simulink model "ADCS_onOrbit"  (R2024b)
settings: Solver=ode4  StartTime=0.0  StopTime=tspan  FixedStep=baseRate  RelTol=1e-3
values from neighbouring files (symbols this model uses):
  A_list = [10*30; 10*30; 10*10; 10*30; 10*30; 10*10] * 1e-04    [adcsInitializer.m]
  A_m = eye(3)    [adcsInitializer.m]
  A_w = eye(3)    [adcsInitializer.m]
  CD = 2.3    [adcsInitializer.m]
  COP = [xAxis/2   0          0 ... (first row only)    [adcsInitializer.m]
  dt = 1    [adcsInitializer.m]
  dYear = decyear(YYYY,MM,DD)    [adcsInitializer.m]
  eta = 0.3    [adcsInitializer.m]
  J_body = [ I_xx  I_xy  I_xz ... (first row only)    [adcsInitializer.m]
  JD0 = juliandate(YYYY,MM,DD,HH,MIN,SEC)    [adcsInitializer.m]
  m = 4    [adcsInitializer.m]
  mag_moment = [0.005; 0.005; 0.005]    [adcsInitializer.m]
  mode = mode(:)    [generateOutput.m]
  mu = 398600.4418    [adcsInitializer.m]    (also in montecarlo.m = mean(W,2))
  n_list = [1 0 0; 0 1 0; 0 0 1; -1 0 0; 0 -1 0; 0 0 -1]    [adcsInitializer.m]
  p = 0.00000451    (= 4.51e-06)    [adcsInitializer.m]
  R = blkdiag(sigma_S^2*eye(3), sigma_B^2*eye(3))    [adcsInitializer.m]
  rE = 6378.14    [adcsInitializer.m]
  sigma_b = deg2rad(0.04)/3600    [adcsInitializer.m]
  sigma_B = 0.001    [adcsInitializer.m]
  sigma_g = deg2rad(0.1)/sqrt(3600)    [adcsInitializer.m]
  sigma_S = deg2rad(0.01)    [adcsInitializer.m]
  T = 1    [adcsInitializer.m]
  wE = [0 0 15.04*(pi/180)*(1/3600)]    [adcsInitializer.m]
  wW_1 = 0    [adcsInitializer.m]
  wW_2 = 0    [adcsInitializer.m]
  wW_3 = 0    [adcsInitializer.m]
undefined symbols (not defined in the file or in its folder): DiscIntNeverNeededParam, J_wheels, K_d, K_p, K_w, n, period, q1_ini, q2_ini, q3_ini, q4_ini, r_I_ini, truevals, useFilter, v_I_ini, wB_1, wB_2, wB_3
libraries: simulink_extras x15, matrix_library x3
(part 2 of 2)

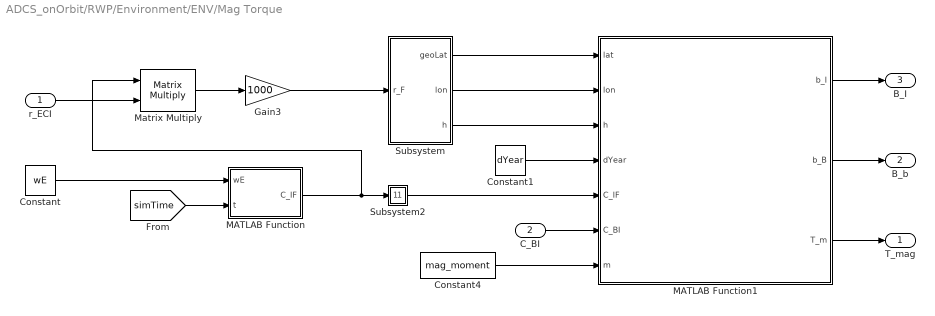
== system ADCS_onOrbit/RWP/Environment/ENV/Mag Torque ==
  r_ECI : Inport
  C_BI : Inport  Port=2
  Constant : Constant  Value=wE
  Constant1 : Constant  Value=dYear
  Constant4 : Constant  Value=mag_moment
  Gain3 : Gain  Gain=1000
  MATLAB Function : MATLAB Function  TreatAsAtomicUnit=on
  MATLAB Function1 : MATLAB Function  TreatAsAtomicUnit=on
  Matrix Multiply : Product  Multiplication=Matrix(*)
  Subsystem : Subsystem
  Subsystem2 : Subsystem
  T_mag : Outport
  B_b : Outport  Port=2
  B_I : Outport  Port=3
  wires:
  C_BI/1 -> MATLAB Function1/6(C_BI)
  Matrix Multiply/1 -> Gain3/1
  r_ECI/1 -> Matrix Multiply/2
  MATLAB Function/1(C_IF) -> Matrix Multiply/1, Subsystem2/1(In1)
  Constant/1 -> MATLAB Function/1(wE)
  [simTime] -> MATLAB Function/2(t)
  Subsystem/1(geoLat) -> MATLAB Function1/1(lat)
  Subsystem/2(lon) -> MATLAB Function1/2(lon)
  Constant1/1 -> MATLAB Function1/4(dYear)
  Constant4/1 -> MATLAB Function1/7(m)
  MATLAB Function1/1(b_I) -> B_I/1
  MATLAB Function1/2(b_B) -> B_b/1
  MATLAB Function1/3(T_m) -> T_mag/1
  Subsystem2/1(Out1) -> MATLAB Function1/5(C_IF)
  Gain3/1 -> Subsystem/1(r_F)
  Subsystem/3(h) -> MATLAB Function1/3(h)

== system ADCS_onOrbit/RWP/Environment/ENV/Solar Radiation Pressure ==
  C_BI : Inport
  s : Inport  Port=2
  MATLAB Function2 : MATLAB Function  TreatAsAtomicUnit=on
  T_SRP : Outport
  wires:
  MATLAB Function2/1(T_SRP) -> T_SRP/1
  C_BI/1 -> MATLAB Function2/2(C_BI)
  s/1 -> MATLAB Function2/1(r_sun)
  [inEclipse] -> MATLAB Function2/3(inEclipse)

== system ADCS_onOrbit/RWP/Environment/ENV/Mag Torque/Subsystem ==
  r_F : Inport
  Constant2 : Constant  Value=rE
  Gain : Gain  Gain=1000
  Geocentric to Geodetic Latitude : Geoc2Geod
  MATLAB Function2 : MATLAB Function  TreatAsAtomicUnit=on
  Scope : Scope
  geoLat : Outport
  lon : Outport  Port=2
  h : Outport  Port=3
  wires:
  MATLAB Function2/2(lon) -> lon/1
  Constant2/1 -> Gain/1, MATLAB Function2/2(rE)
  r_F/1 -> MATLAB Function2/1(r_F)
  MATLAB Function2/1(lat) -> Geocentric to Geodetic Latitude/1
  Geocentric to Geodetic Latitude/1 -> geoLat/1
  MATLAB Function2/3(h) -> Scope/1, h/1
  Gain/1 -> Geocentric to Geodetic Latitude/2

== system ADCS_onOrbit/RWP/Environment/ENV/Mag Torque/Subsystem2 ==
  In1 : Inport
  Out1 : Outport
  tag scope: C_IF=global
  wires:
  In1/1 -> [C_IF], Out1/1

== matlab function ADCS_onOrbit/GNC/Guidance/Error/MATLAB Function ==
  settings: updateMethod=DISCRETE  sampleTime=baseRate
  data: q_error input; theta_e output
function theta_e = pointing_error(q_error)

    q_error = q_error/norm(q_error);
    q4 = q_error(4);
    
    theta_e = rad2deg(2*acos(q4));

end

== matlab function ADCS_onOrbit/GNC/Guidance/Subsystem3/MATLAB Function1 ==
  data: q input; roll output; pitch output; yaw output
function [roll, pitch, yaw] = fcn(q)

    E = q(1:3);
    n = q(4);

    C_BI = (n^2 - E'*E) * eye(3) + 2*(E*E') - 2*n*skew(E);

    roll    = atan2(C_BI(2,3),C_BI(3,3));
    pitch   = -asin(C_BI(1,3));
    yaw     = atan2(C_BI(1,2),C_BI(1,1)); 


end

== matlab function ADCS_onOrbit/RWP/Orbit Propator/MATLAB Function2 ==
  settings: updateMethod=DISCRETE  sampleTime=baseRate
  data: r_S input; s output
function s = fcn(r_S)

s = r_S/norm(r_S);

== matlab function ADCS_onOrbit/RWP/Environment/ENV/Mag Torque/MATLAB Function1 ==
  settings: updateMethod=DISCRETE  sampleTime=1
  data: lat input; b_I output; lon input; h input; dYear input; C_IF input; C_BI input; m input; b_B output; T_m output
function [b_I, b_B, T_m] = fcn(lat, lon, h, dYear, C_IF, C_BI, m)

    coder.extrinsic('wrldmagm');
    
    % dYear = 2025.0;
    b = zeros(3,1);
    lat_geo = lat;

    m_skew = skew(m);
    
    % World Magnetic Model
    % [b, H, DEC, DIP, F] = wrldmagm(h, lat, lon, dYear,'Custom','WMM2025.COF');
    [b, H, DEC, DIP, F] = wrldmagm(h, lat, lon, dYear, 2020);

    % Conversion to go from NED to ECEF
    sLat = sind(lat_geo);
    cLat = cosd(lat_geo);

    sLon = sind(lon);
    cLon = cosd(lon);
 
    C_FN = [-sLat*cLon -sLat*sLon cLat; -sLon cLon 0; -cLat*cLon -cLat*sLon -sLat]';
    b_ECEF = C_FN * b;

    % Going from ECEF to ECI
    b_I = C_IF * b_ECEF;

    % Conversion to Body Frame
    b_B = C_BI * b_I;

    % Magnetic Torque
    T_m = m_skew * b_B * 1e-09;

end

== matlab function ADCS_onOrbit/SENS/Magnetometer/MATLAB Function ==
  settings: updateMethod=DISCRETE  sampleTime=baseRate
  data: meas input; y output; true input; set input
function y = fcn(meas, true, set)

y = (set ~= 0) * true + (set == 0) * meas;

== matlab function ADCS_onOrbit/SENS/Sun Sensor/MATLAB Function ==
  settings: updateMethod=DISCRETE  sampleTime=baseRate
  data: meas input; y output; true input; set input
function y = fcn(meas, true, set)

y = (set ~= 0) * true + (set == 0) * meas;

== matlab function ADCS_onOrbit/RWP/Nonlinear Spacecraft/Spacecraft Dynamics/MATLAB Function1 ==
  settings: updateMethod=DISCRETE  sampleTime=baseRate
  data: h_tot input; T_b input; h_tot_dot output; h_w input; w_b output; J_body parameter; A_w parameter
function [h_tot_dot, w_b] = dynamics(h_tot, T_b, h_w, J_body, A_w)

% Nimish Dhawan 2025

% T_b : net body torque (ext + MTQ - wheel torque on body)      [3x1]
% J     : body inertia                                          [3x3]
% A_w   : wheel axis matrix (columns = wheel axes, body frame)  [3x3]
% h_w   : wheel angular momentum                                [3x1]
% h_tot : current total angular momentum of SC (state)          [3x1]

% ---- omega from momentum ----
w_b = J_body \ (h_tot - A_w * h_w);       

% ---- h_tot dynamics ----
h_tot_dot = T_b - skew(w_b) * h_tot;

end

== matlab function ADCS_onOrbit/RWP/Nonlinear Spacecraft/Spacecraft Kinematics/MATLAB Function1 ==
  settings: updateMethod=DISCRETE  sampleTime=baseRate
  data: q input; q_dot output; w input
function q_dot = kinematics(q, w)

% Nimish Dhawan 2025
% Input: 
% q = quaternion (4x1) [scalar last]
% w = angular velocity of s/c (3x1) [SBF]

E   = q(1:3);
Eta = q(4);

E_dot   = 0.5 * (Eta*eye(3) + skew(E)) * w;
Eta_dot = -0.5 * (E' * w); 

q_dot = [E_dot; Eta_dot];

end

== matlab function ADCS_onOrbit/RWP/Nonlinear Spacecraft/Spacecraft Kinematics/Quaternion Normalize1 ==
  settings: updateMethod=DISCRETE  sampleTime=baseRate
  data: q input; q_norm output
function q_norm = q_normalize(q)

q_norm = q/norm(q);

== matlab function ADCS_onOrbit/RWP/Orbit Propator/Two Body/MATLAB Function1 ==
  settings: updateMethod=DISCRETE  sampleTime=baseRate
  data: r_I input; a_I output; mu input
function a_I = fcn(r_I, mu)

a_I = r_I .* (-mu / (norm(r_I)^3));

end

== matlab function ADCS_onOrbit/RWP/Orbit Propator/Two Body/MATLAB Function3 ==
  settings: updateMethod=DISCRETE  sampleTime=baseRate
  data: r input; a_j2 output; mu input; rE input
function a_j2 = J2_perturbation(r, mu, rE)

    J2 = 1.08263e-3;

    x = r(1); y = r(2); z = r(3);
    r_norm = norm(r);

    factor = -(3/2) * J2 * mu * rE^2 / r_norm^5;
    zx2_r2 = 5*z^2 / r_norm^2;

    a_j2 = factor * [
        x * (1 - zx2_r2);
        y * (1 - zx2_r2);
        z * (3 - zx2_r2)
    ];
    
end

== matlab function ADCS_onOrbit/RWP/Orbit Propator/MATLAB Function ==
  settings: updateMethod=DISCRETE  sampleTime=baseRate
  data: q input; C_BI output
function C_BI = QUAT2DCM(q)

% Nimish Dhawan
% 2025

%%%%%%%%%%%%%%%%%%%%%%%%%%%%%%%%%%%%%%%%%%%%%%%%%%%%%%%%%%%%%%%%%%%%%%%%%
% Input(s)
%%%%%%%%%%%%%%%%%%%%%%%%%%%%%%%%%%%%%%%%%%%%%%%%%%%%%%%%%%%%%%%%%%%%%%%%%
% q (4x1): Quaternion

%%%%%%%%%%%%%%%%%%%%%%%%%%%%%%%%%%%%%%%%%%%%%%%%%%%%%%%%%%%%%%%%%%%%%%%%%
% Output(s)
%%%%%%%%%%%%%%%%%%%%%%%%%%%%%%%%%%%%%%%%%%%%%%%%%%%%%%%%%%%%%%%%%%%%%%%%%
% C_BI (3x3): Rotation matrix to go from ECI to Body Fixed Frame

E = q(1:3);
Eta = q(4);

C_BI = (Eta^2-E'*E)*eye(3) + 2*(E*E') - 2*Eta*skew(E);

== matlab function ADCS_onOrbit/ACT/Wheels + Magnetorquers/Wheel 1/MATLAB Function1 ==
  settings: updateMethod=DISCRETE  sampleTime=baseRate
  data: h_wi output; w_wi output; J_w input; h_w input; wB input; A_w input
function [h_wi, w_wi] = fcn(J_w, h_w, wB, A_w)

% Nimish Dhawan 2025

i       = 1;      % Wheel No.


J_inv   = 1 / J_w;
Aw_i    = A_w(:,i);
h_wi    = h_w ;

w_wi = (J_inv*h_wi) * Aw_i;

end

== matlab function ADCS_onOrbit/ACT/Wheels + Magnetorquers/Wheel 2/MATLAB Function1 ==
  settings: updateMethod=DISCRETE  sampleTime=baseRate
  data: h_wi output; w_wi output; J_w input; h_w input; wB input; A_w input
function [h_wi, w_wi] = fcn(J_w, h_w, wB, A_w)

% Nimish Dhawan 2025

i       = 2;      % Wheel No.

J_inv   = 1 / J_w;
Aw_i    = [A_w(:,i)];
h_wi    = h_w ;

w_wi = (J_inv*h_wi) * Aw_i;

end

== matlab function ADCS_onOrbit/RWP/Environment/MATLAB Function ==
  settings: updateMethod=DISCRETE  sampleTime=baseRate
  data: u input; y output
function y = magnitude(u)

y = norm(u);

== matlab function ADCS_onOrbit/ACT/Wheels + Magnetorquers/Wheel 3/MATLAB Function1 ==
  settings: updateMethod=DISCRETE  sampleTime=baseRate
  data: h_wi output; w_wi output; J_w input; h_w input; wB input; A_w input
function [h_wi, w_wi] = fcn(J_w, h_w, wB, A_w)

% Nimish Dhawan 2025

i       = 3;      % Wheel No.

J_inv   = 1 / J_w;
Aw_i    = [A_w(:,i)];
h_wi    = h_w ;

w_wi = (J_inv*h_wi) * Aw_i;

end

== matlab function ADCS_onOrbit/RWP/Environment/ENV/Gravity Gradient/MATLAB Function3 ==
  settings: updateMethod=DISCRETE  sampleTime=1
  data: r_I input; J input; mu input; C_BI input; T_g output
function T_g = fcn(r_I, J, mu, C_BI)

r_B = C_BI * r_I;
r = norm(r_I);

T_g = (3*mu/r^5) * skew(r_B) * J * r_B;

== matlab function ADCS_onOrbit/ACT/Wheels + Magnetorquers/Reaction Wheel Power/MATLAB Function3 ==
  data: Tc input; Prw output; h_W input; Ptotal output; P_pre input
function [Prw, Ptotal]= fcn(Tc, h_W, P_pre)

% Nimish Dhawan
% Reaction wheel power consumption as given in "Comarison of Control Moment
% Gyros and Reaction Wheels for Small Earth-Observing Satellites


% Eq. 3
alpha = 0.47;     % empirical exponent
k2    = 4.51;     % empirical coeff

Prw = 1000.*abs(Tc) + k2.*(abs(h_W).^(alpha));   % per-wheel power [W]
Ptotal = (P_pre + Prw); 

end

== matlab function ADCS_onOrbit/GNC/Guidance/Attitude Guidance ==
  settings: updateMethod=DISCRETE  sampleTime=baseRate
  data: q_prev input; opMode input; s_i input; r input; v input; C_IF input; q output; w output; mode output; n parameter; rE parameter; CQI output
function [q, w, mode, CQI] = fcn(q_prev, opMode, s_i, r, v, C_IF, n, rE)


    option = opMode;
    q = zeros(4,1);
    w = zeros(3,1);
    CQI = zeros(3,3);
    mode = 0;

    % Manual override modes
    % For mission mode, detumble mode, desaturation mode and safemode
    if option ~= 1 && option ~= 2 && option ~= 3
        [q, w] = nadir(r, v, n, q_prev);
        mode = 0;

    % For comms mode
    elseif option == 3
        [q, w] = gnd(C_IF, rE, r, v, q_prev);
       
    % Idle mode
    elseif option == 1
        [q, w] = sun(s_i);
        mode = 1;
    end

    CQI = rpy(r, v);
end

%%
function [q_nadir, w_nadir] = nadir(r, v, n, q_prev)

    C_BI = rpy(r, v);

    q = CBI2quat(C_BI');
    q_nadir = continuity(q, q_prev);
    w_nadir = [0; -n; 0];
end

%%
function [q_sun, w_sun] = sun(s_i)
    % coder.extrinsic('dcm2quat');
    % Ecliptic north pole
    epsilon = deg2rad(23.44);  % Obliquity of the ecliptic
    n_ecl = [0; -sin(epsilon); cos(epsilon)];

    x_b = s_i / norm(s_i);
    z_b = n_ecl - dot(n_ecl, x_b) * x_b; % Gram-Schmidt orthogonalization
    z_b = z_b / norm(z_b); 
    if dot(z_b, n_ecl) < 0
        z_b = -z_b; 
    end
    y_b = cross(z_b, x_b);
    
    C1 = [x_b y_b z_b];   

    theta = deg2rad(45);

    Rz = [cos(theta), sin(theta), 0;
          -sin(theta), cos(theta), 0;
          0,           0,          1];
    
    C_BI = C1 * Rz;
    q = r2quat(C_BI);
    % q_sun = continuity(q, q_prev);
    % q_sun = [q(2:4);q(1)];
    q_sun = q;
    w_sun = [0;0;0];

end

%%
function [q_gnd, w_gnd] = gnd(C_IF, rE, r, v, q_prev)
    dt = 1;

    target_lat = 45.3848;
    target_lon = - 75.6974;

    lat = deg2rad(target_lat);
    lon = deg2rad(target_lon);
    
    x_F= rE * cos(lat) * cos(lon);
    y_F= rE * cos(lat) * sin(lon);
    z_F= rE * sin(lat);
    
    r_target_I = C_IF * [x_F; y_F; z_F];
    los = r - r_target_I;
    los = los / norm(los);
    
    z_orb = los;

    y_orb = cross(v, r) / norm(cross(v,r)); % orbit normal
    y_orb = y_orb / norm(y_orb);

    x_orb = cross(y_orb, z_orb); 
    x_orb = x_orb / norm(x_orb);
    
    C_BI = [x_orb, y_orb, z_orb];

    q = CBI2quat(C_BI);
    q_gnd = continuity(q, q_prev);
    q_dot = (q_gnd - q_prev)/dt;
    E = q_gnd(1:3);
    n = q_gnd(4);
    Edot = q_dot(1:3);
    w_gnd = (2/n) * (n^2*eye(3) - n*skew(E) + (E*E'))*Edot; 
end

%%
function CQI = rpy(r, v)
    z_orb = - r / norm(r);                  % nadir
    y_orb = cross(v, r) / norm(cross(v,r)); % orbit normal
    y_orb = y_orb / norm(y_orb);

    x_orb = cross(y_orb, z_orb); 
    x_orb = x_orb / norm(x_orb);

    CQI = [x_orb, y_orb, z_orb]';
end

%%
function q = r2quat(DCM)
    A = DCM;
    q = zeros(4,1); % [q1; q2; q3; q4] — vector-first

    tr = trace(A);

    if tr > 0
        S = sqrt(tr + 1.0) * 2; % S = 4*q4
        q(4) = 0.25 * S;
        q(1) = (A(3,2) - A(2,3)) / S;
        q(2) = (A(1,3) - A(3,1)) / S;
        q(3) = (A(2,1) - A(1,2)) / S;
    elseif (A(1,1) > A(2,2)) && (A(1,1) > A(3,3))
        S = sqrt(1.0 + A(1,1) - A(2,2) - A(3,3)) * 2; % S = 4*q1
        q(1) = 0.25 * S;
        q(2) = (A(1,2) + A(2,1)) / S;
        q(3) = (A(1,3) + A(3,1)) / S;
        q(4) = (A(3,2) - A(2,3)) / S;
    elseif (A(2,2) > A(3,3))
        S = sqrt(1.0 + A(2,2) - A(1,1) - A(3,3)) * 2; % S = 4*q2
        q(1) = (A(1,2) + A(2,1)) / S;
        q(2) = 0.25 * S;
        q(3) = (A(2,3) + A(3,2)) / S;
        q(4) = (A(1,3) - A(3,1)) / S;
    else
        S = sqrt(1.0 + A(3,3) - A(1,1) - A(2,2)) * 2; % S = 4*q3
        q(1) = (A(1,3) + A(3,1)) / S;
        q(2) = (A(2,3) + A(3,2)) / S;
        q(3) = 0.25 * S;
        q(4) = (A(2,1) - A(1,2)) / S;
    end

    q = q / norm(q); % normalize
end

== matlab function ADCS_onOrbit/RWP/Environment/ENV/Drag/Atmosphere Model ==
  settings: updateMethod=DISCRETE  sampleTime=baseRate
  data: rho output; r input; rE input
function rho = atmosphere(r, rE)

    z = norm(r)-rE;        % Altitude (km) 
    
    if 400 <= z && z < 450
        rho0 = 3.275e-12;
        h0   = 400;
        H    = 58.515;
    elseif 450 <= z && z < 500
        rho0 = 1.585e-12;   % kg/m³
        h0   = 450;   % km
        H    = 60.828;  % km
    elseif 500 <= z && z < 600
        rho0 = 6.967e-13;   % kg/m³
        h0   = 500;   % km
        H    = 63.822;  % km
    elseif 600 <= z && z < 700
        rho0 = 1.454e-13;
        h0   = 600;
        H    = 71.835;
    elseif 700 <= z && z < 800
        rho0 = 3.614e-14;
        h0   = 700;
        H    = 88.667;
    else
        rho0 = 1.170e-14;
        h0   = 800;
        H    = 124.64;
    end

    rho = rho0 * exp(-(z-h0)/H);    % in kg/m³

end

== matlab function ADCS_onOrbit/RWP/Environment/ENV/Drag/Drag Torque ==
  settings: updateMethod=DISCRETE  sampleTime=baseRate
  data: v_RI input; C_BI input; A_list input; n_list input; COP_B input; CD input; T_atm output; rho input; a_drag output; m input
function [T_atm, a_drag] = drag_torque(v_RI, C_BI, A_list, n_list, COP_B, CD, rho, m)

    v_RI_hat = v_RI / norm(v_RI);     
    v_RI_mag = norm(v_RI);            
    T_atm = [0; 0; 0];
    F_drag = [0; 0; 0];
    a_drag = [0; 0; 0];

    for k = 1:length(A_list)
        n_k = n_list(k, :).';         
        A_k = A_list(k);              

        cos_alpha_k = dot(n_k, C_BI * v_RI_hat);

        if cos_alpha_k > 0
            F_k = - 0.5 * rho * CD * A_k * v_RI_mag^2 * cos_alpha_k * v_RI_hat;
        else 
            F_k = [0; 0; 0];
        end
        F_drag = F_drag + F_k;
        a_drag = F_drag/m;

        F_k_B = C_BI * F_k;
        COP_B_k = COP_B(k, :).';
        T_k = cross(COP_B_k, F_k_B);
        T_atm = T_atm + T_k;
    end

end

== matlab function ADCS_onOrbit/TTC/RES/MATLAB Function ==
  data: u input; y output
function y = magnitude(u)

y = norm(u);

== matlab function ADCS_onOrbit/RWP/Environment/ENV/Drag/skew symmetric ==
  settings: updateMethod=DISCRETE  sampleTime=baseRate
  data: M input; skew output
function skew = skew_matrix(M)

    skew = [0 M(3) -M(2)
            -M(3) 0 M(1)
            M(2) -M(1) 0];

end

== matlab function ADCS_onOrbit/GNC/Navigation/MEKF/MEKF ==
  settings: updateMethod=DISCRETE  sampleTime=baseRate
  data: x_pre input; w_meas input; q_triad input; y input; useFilter input; q_est output; b_est output; P_pre input; P_est output; sigma_g parameter; sigma_b parameter; dt parameter; R parameter
function [q_est, b_est, P_est] = est(x_pre, w_meas, q_triad, y, useFilter , P_pre, sigma_g, sigma_b, ...
dt, R)

q_pre = x_pre(1:4);
b_pre = x_pre(5:7);

% Simulink acting out badly and thinking w_meas is 9x1
b_pre = reshape(b_pre, [3,1]);
w_meas = w_meas(1:3);   

s_I = y(1:3);
s_B = y(7:9);
b_I = y(4:6);
b_B = y(10:12);

if useFilter ~= 0
    [q_est, b_est, P_est] = mekf(q_pre, w_meas, b_pre, dt, s_I, ...
                                b_I, s_B, b_B, R, sigma_g, sigma_b, P_pre);
else
    q_est = q_triad;
    b_est = zeros(3,1);
    P_est = zeros(6,6);
end

end

== matlab function ADCS_onOrbit/RWP/Orbit Propator/Eclipse Detection/MATLAB Function3 ==
  settings: updateMethod=DISCRETE  sampleTime=baseRate
  data: R_s input; eclipse_entry output; r_sat input; r_E input; was_in_eclipse input; eclipse_exit output; is_in_eclipse output
function [eclipse_entry, eclipse_exit, is_in_eclipse] = fcn(R_s, r_sat, r_E, was_in_eclipse)

    % Convert input to numeric (if it came in as logical)
    if was_in_eclipse
        was = 1;
    else
        was = 0;
    end

    % Normalize sun vector
    s_hat = R_s / norm(R_s);

    % Projection of satellite position onto sun vector
    proj = dot(r_sat, s_hat);
    closest_point = proj * s_hat;

    % Perpendicular distance from Earth center to Sun-sat line
    d = norm(r_sat - closest_point);

    % Check if satellite is in eclipse
    if (d < r_E) && (proj < 0)
        is_in_eclipse = 1;
    else
        is_in_eclipse = 0;
    end

    % Detect eclipse entry
    if (was == 0) && (is_in_eclipse == 1)
        eclipse_entry = 1;
    else
        eclipse_entry = 0;
    end

    % Detect eclipse exit
    if (was == 1) && (is_in_eclipse == 0)
        eclipse_exit = 1;
    else
        eclipse_exit = 0;
    end

end

== matlab function ADCS_onOrbit/SENS/Gyroscope/MATLAB Function1 ==
  settings: updateMethod=DISCRETE  sampleTime=baseRate
  data: w_sc input; w_meas output; bias input; noise input
function w_meas = fcn(w_sc, bias, noise)

rand_w = noise .* ones(3,1);
bias   = bias .* ones(3,1);

w_meas = w_sc + bias + rand_w;

== matlab function ADCS_onOrbit/GNC/Navigation/Subsystem1/MATLAB Function2 ==
  data: q input; roll output; pitch output; yaw output; C_QI input
function [roll, pitch, yaw] = fcn(q, C_QI)

    E = q(1:3);
    n = q(4);

    C_BI = (n^2 - E'*E) * eye(3) + 2*(E*E') - 2*n*skew(E);
    C_BQ = C_BI * C_QI';
    
    roll    = atan2(C_BQ(2,3),C_BQ(3,3));
    pitch   = -asin(C_BQ(1,3));
    yaw     = atan2(C_BQ(1,2),C_BQ(1,1));

end

== matlab function ADCS_onOrbit/SENS/Gyroscope/MATLAB Function2 ==
  data: true input; meas input; y output; set input
function y = fcn(true, meas, set)

y = (set ~= 0) * true + (set == 0) * meas;

== matlab function ADCS_onOrbit/RWP/Environment/ENV/Mag Torque/Subsystem/MATLAB Function2 ==
  data: r_F input; lat output; lon output; rE input; h output
function [lat, lon, h] = fcn(r_F, rE)

r = norm(r_F);

lat = asind(r_F(3)/r);

if r_F(2)/r > 0
    lon = acosd(r_F(1)/(r*cosd(lat)));
else
    lon = 360 - acosd(r_F(1)/(r*cosd(lat)));
end

h = r - rE*1000;

end

== matlab function ADCS_onOrbit/ACT/Wheels + Magnetorquers/MATLAB Function ==
  settings: updateMethod=DISCRETE  sampleTime=baseRate
  data: T_c input; T_cmd output; wheelsEnabled input
function T_cmd = fcn(T_c, wheelsEnabled)

if wheelsEnabled == 1
    T_cmd = T_c;
else
    T_cmd = [0; 0; 0];
end

end

== matlab function ADCS_onOrbit/RWP/Environment/ENV/Mag Torque/MATLAB Function ==
  data: wE input; C_IF output; t input
function C_IF = fcn(wE, t)

    theta = wE(3) * t;

    C_IF = [cos(theta) sin(theta) 0; -sin(theta) cos(theta) 0; 0 0 1]';

end

== matlab function ADCS_onOrbit/RWP/Environment/ENV/Solar Radiation Pressure/MATLAB Function2 ==
  settings: updateMethod=DISCRETE  sampleTime=baseRate
  data: r_sun input; T_SRP output; C_BI input; inEclipse input; p parameter; eta parameter; A_list parameter; n_list parameter; COP parameter
function T_SRP = srpT(r_sun, C_BI, inEclipse, p, eta, A_list, n_list, COP)

    T_SRP = [0; 0; 0];
    r_sun = r_sun(:);  

    for k = 1:length(A_list)
        n_k = n_list(k, :)';          % column vector (3x1)
        A_k = A_list(k);              % scalar area

        cos_alpha_k = dot(n_k, C_BI * r_sun);  

        if cos_alpha_k > 0 && inEclipse == 0
            F_srp_k = -p * A_k * eta * cos_alpha_k * r_sun;  
        else
            F_srp_k = [0; 0; 0];
        end

        F_srp_k_B = C_BI * F_srp_k;
        COP_k = COP(k, :)';
        T_SRP_k = cross(COP_k, F_srp_k_B);

        T_SRP = T_SRP + T_SRP_k;
    end

end

== matlab function ADCS_onOrbit/GNC/Navigation/TRIAD Determination/MATLAB Function1 ==
  settings: updateMethod=DISCRETE  sampleTime=baseRate
  data: s_I input; q_triad output; m_I input; s_b input; m_b input; q_prev input
function q_triad = fcn(s_I, m_I, s_b, m_b, q_prev)

% Normalizing vectors
sI = s_I/norm(s_I);
sB = s_b/norm(s_b);
mI = m_I/norm(m_I);
mB = m_b/norm(m_b);

% Determining M_I 
r1 = sI;
r2 = skew(sI)*mI/norm(skew(sI)*mI);
r3 = skew(r1) * r2;
MI = [r1, r2, r3];

% Determining M_B
s1 = sB;
s2 = skew(sB)*mB/norm(skew(sB)*mB);
s3 = skew(s1) * s2;

MB = [s1, s2, s3]; 

C_BI = MB * MI';

q = CBI2quat(C_BI);
q_triad = continuity(q, q_prev);

end

%%

== matlab function ADCS_onOrbit/SENS/Gyroscope/MATLAB Function ==
  settings: updateMethod=DISCRETE  sampleTime=baseRate
  data: biasDot output; noise input
function biasDot = fcn(noise)

bias_noise = noise.*[1;1;1];

biasDot = bias_noise;

== matlab function ADCS_onOrbit/GNC/Control/Controller ==
  settings: updateMethod=DISCRETE  sampleTime=baseRate
  data: opMode input; t input; T_w output; B_meas input; w input; q_error input; w_error input; h_w input; M output; period parameter; J_body parameter; K_p parameter; K_d parameter; K_w parameter; m_pre input; m output
function [T_w, M, m] = fcn(opMode ,t, B_meas, w, q_error, w_error, h_w, period, J_body, K_p, K_d, K_w, m_pre)

T_w = [0; 0; 0];
M = [0; 0; 0];
w_skew = skew(w);

% Modified PD control
if opMode ~= 4 && opMode ~= 5 && opMode ~= 6 && opMode ~= 7 && opMode ~= 8

    % Gain Scheduling
    theta_e = 2*atan2(norm(q_error(1:3)), q_error(4));
    wr = norm(w_error);

    Kd0 = diag(K_d*ones(3,1));
    Kp0 = diag(K_p*ones(3,1));

    % Kd0 = diag([0.01, 0.025, 0.01]);
    % Kp0 = diag([0.000125/2, 0.000125, 0.000125/2])./2;

    e1 = deg2rad(1.0);
    e2 = deg2rad(3.0);
    w1 = deg2rad(0.05);
    w2 = deg2rad(0.1);

    % alpha_p = (theta_e < e1)*0.6 + (theta_e >= e1 && theta_e < e2)*5.0 + (theta_e >= e2)*1.6;
    % alpha_d = (wr < w1)*0.9 + (wr >= w1 && wr < w2)*1.2 + (wr >= w2)*1.6;

    alpha_p = (theta_e < e1)*0.6 + (theta_e >= e1 && theta_e < e2 && opMode == 0)*5.0 + ...
                (theta_e >= e1 && theta_e < e2 && opMode == 1)*0.2 + (theta_e >= e2)*1;
    alpha_d = (wr < w1)*0.9 + (wr >= w1 && wr < w2)*1.2 + (wr >= w2)*2;

    if wr >= w2
        alpha_p = 0.7*alpha_p;
        alpha_d = 1.3*alpha_d;
    end

    alpha_p = min(max(alpha_p,0.0),2.5);
    alpha_d = min(max(alpha_d,0.5),3.0);

    K_p = alpha_p*Kp0;
    K_d = alpha_d*Kd0;
        
    % K_d = diag([0.01, 0.025, 0.01]);
    % K_p = diag([0.000125/2, 0.000125, 0.000125/2])./2;

    % Control algorithm
    T_w = w_skew * J_body * w + K_p * eye(3) * q_error(1:3) + K_d * eye(3) * w_error;
    m = m_pre;

% B-dot 
elseif opMode == 8
    M = -K_w * skew(B_meas) * w;
    m = m_pre;

% No control - Safe mode and LEOP
elseif opMode == 6 || opMode == 7
    T_w = [0; 0; 0];
    M = [0; 0; 0];
    m = m_pre;

% Desaturation (incomplete)
elseif opMode == 5
    % Trigger for dumping
    if t < (12*period) && t > (10*period) % Create a proper autonomous trigger for dumping
        k_desat = -0.0005;
    else
        k_desat = 0;
    end

    % Controller gains
    K_p = 5e-4;
    K_d = 5e-05;
    
    % Desired wheel momentum [h_w1; h_w2; h_w3]
    h_wn = [0; 0; 0];
    B2 = norm(B_meas)^2;

    % Control algorithm
    T_ctrl = w_skew * J_body * w + K_p * eye(3) * q_error(1:3) + K_d * eye(3) * w_error;
    M_dump = (k_desat/B2) * (cross(B_meas, (h_w - h_wn))); 
    % T_dump = cross(M_dump, B_meas);

    T_w = T_ctrl;
    M = M_dump;
    % T_mag = T_dump;
    % 
    % M = (1/B2) * cross(B_meas, T_mag);
    m = m_pre;

% Simple Bdot Detumble (works)
elseif opMode == 4
    [T_w, M, m] = detumble(w, J_body, w_skew, q_error, K_p, K_d, K_w, w_error, B_meas, m_pre);

else
    % unknown opMode (or NaN) -> safe outputs
    T_w = [0;0;0];
    M   = [0;0;0];
    m   = 0;

end

end

%%
function [T_w, M, m] = detumble(w, J_body, w_skew, q_error, K_p, K_d, K_w, w_error, B_meas, m_pre)
% Latch doesnt work :(
    wr = norm(w);
    if m_pre ~= 1
        Kw0 = K_w;
        alpha = (wr > deg2rad(1)) * 5 + (wr <= deg2rad(1)) * 10;
        Kw = alpha*Kw0;
        M = - Kw * skew(B_meas) * w;
        T_w = [0; 0; 0];
        if wr < 0.01
            m = 1;
        else
            m = 0; 
        end
    elseif m_pre == 1  %wr < deg2rad(0.5) &&
        T_w = w_skew * J_body * w + K_p * eye(3) * q_error(1:3) + K_d * eye(3) * w_error;
        M = [0; 0; 0]; 
        m = 1;
    else
        T_w = [0; 0; 0];
        M = [0; 0; 0]; 
        m = 0;
    end

end

== matlab function ADCS_onOrbit/ACT/Wheels + Magnetorquers/Magnetorquer 1/skew symmetric ==
  data: M input; skew output
function skew = skew_matrix(M)

    skew = [0 M(3) -M(2)
            -M(3) 0 M(1)
            M(2) -M(1) 0];

end

== matlab function ADCS_onOrbit/ACT/Wheels + Magnetorquers/Magnetorquer 2/skew symmetric ==
  data: M input; skew output
function skew = skew_matrix(M)

    skew = [0 M(3) -M(2)
            -M(3) 0 M(1)
            M(2) -M(1) 0];

end

== matlab function ADCS_onOrbit/RWP/Nonlinear Spacecraft/Subsystem/MATLAB Function2 ==
  data: q input; roll output; pitch output; yaw output; C_QI input
function [roll, pitch, yaw] = fcn(q, C_QI)

    E = q(1:3);
    n = q(4);

    C_BI = (n^2 - E'*E) * eye(3) + 2*(E*E') - 2*n*skew(E);
    C_BQ = C_BI * C_QI';
    
    roll    = atan2(C_BQ(2,3),C_BQ(3,3));
    pitch   = -asin(C_BQ(1,3));
    yaw     = atan2(C_BQ(1,2),C_BQ(1,1));

end

== matlab function ADCS_onOrbit/ACT/Wheels + Magnetorquers/Magnetorquer 3/skew symmetric ==
  data: M input; skew output
function skew = skew_matrix(M)

    skew = [0 M(3) -M(2)
            -M(3) 0 M(1)
            M(2) -M(1) 0];

end

== matlab function ADCS_onOrbit/ACT/Wheels + Magnetorquers/MATLAB Function1 ==
  settings: updateMethod=DISCRETE  sampleTime=baseRate
  data: M_c input; M_cmd output; rodsEnable input
function M_cmd = fcn(M_c, rodsEnable)

if rodsEnable == 1
    M_cmd = M_c;
else
    M_cmd = [0; 0; 0];
end

end

== matlab function ADCS_onOrbit/GNC/Navigation/MATLAB Function ==
  settings: updateMethod=DISCRETE  sampleTime=baseRate
  data: u input; y output
function y = fcn(u)

y = norm(u);

== matlab function ADCS_onOrbit/TTC/MATLAB Function ==
  settings: updateMethod=DISCRETE  sampleTime=baseRate
  data: internal input; mode output; fromTable input; wheelsEnable output; rodsEnable output
function [mode, wheelsEnable, rodsEnable] = fcn(internal, fromTable)

if internal ~= 2
    mode = internal;
    wheelsEnable    = 1;
    rodsEnable      = 1;
else
    mode            = fromTable(1);
    wheelsEnable    = fromTable(3);
    rodsEnable      = fromTable(2);
end

end

== matlab function ADCS_onOrbit/RWP/Orbit Propator/MATLAB Function1 ==
  settings: updateMethod=DISCRETE  sampleTime=baseRate
  data: t input; r_SI output; JD0 input
function r_SI = sun_vector(t, JD0)

    JD = JD0 + 1.157e-05*t;
    TUT = (JD-2451545)/36525;
    mean_long = 280.4606184 + 36000.77005361*TUT;
    mean_anom = 357.5277233 + 35999.0534*TUT;
    obliquity = 23.439291 - 0.0130042*TUT;
    lambda_e = mean_long + 1.914666471 * sind(mean_anom) + 0.019994643 * sind(2*mean_anom);
    r_sun_norm = (1.000140612 - 0.016708617 * cosd(mean_anom) + 0.019994643 * sind(2*mean_anom)) * 149597870.691; % km
    r_SI = r_sun_norm * [cosd(lambda_e); cosd(obliquity) * sind(lambda_e); sind(obliquity) * sind(lambda_e)];

end

== matlab function ADCS_onOrbit/GNC/Navigation/Subsystem/MATLAB Function2 ==
  data: q input; roll output; pitch output; yaw output; C_QI input
function [roll, pitch, yaw] = fcn(q, C_QI)

    E = q(1:3);
    n = q(4);

    C_BI = (n^2 - E'*E) * eye(3) + 2*(E*E') - 2*n*skew(E);
    C_BQ = C_BI * C_QI';
    
    roll    = atan2(C_BQ(2,3),C_BQ(3,3));
    pitch   = -asin(C_BQ(1,3));
    yaw     = atan2(C_BQ(1,2),C_BQ(1,1));

end

== matlab function ADCS_onOrbit/GNC/Guidance/Error/Error Quaternion ==
  settings: updateMethod=DISCRETE  sampleTime=baseRate
  data: q input; delta_q output; q_d input
function delta_q = error_quaternion(q, q_d)
% Nimish Dhawan 2025

    delta_q = zeros(4,1);
    q_d_tilde = zeros(4, 4);

    q_conj = [-q(1:3); q(4)];

    E = q_d(1:3);

    E_skew = skew(E);
    Eta = q_d(4);

    q_d_tilde = [Eta*eye(3)-E_skew, E; -E', Eta];

    delta_q = q_d_tilde * q_conj;

end
